simulink model "Brat_Robotic"  (R2022b)
settings: Solver=VariableStepAuto  StartTime=0.0  StopTime=timp  MaxStep=0.01  RelTol=1e-3
InitFcn:
  | %Elements lengths cm
  |     l1 = 24;
  |     l2 = 24;
  |     l3 = 20;
  |     l4 = 24;
  |     l5 = 10;
  |     l6 = 8;
  |     l7= 7;
  | 
  |     %sim time
  |     %timp=10;
  | 
  |     D1 = input_cupla_1/100;
  |     D2 = input_cupla_2*pi/180;
  |     D3 = input_cupla_3*pi/180;
  |     D4 = input_cupla_4/100;
  |     D5 = input_cupla_5*pi/180;
  |     D6 = input_cupla_6/100;
  |     D7 = input_cupla_7/100;
  | 
  |     %{
  |     D1 = 0.04;
  |     D2 = pi/3;
  |     D3 = -pi/5;
  |     D4 = 0.06;
  |     D5 = pi/8;
  |     D6 = 0.02;
  |     D7 = 0.02;
  | 
  |     prompt="Folositi comenzile default: ";
  |     default = input(prompt);
  | 
  |     if (default == 0)
  | 
  | 
  |     prompt="Cupla 1 (translatie):";
  |     D1 = input(prompt);
  |     prompt="Cupla 2 (rotatie):";
  |     D2 = input(prompt);
  |     prompt="Cupla 3 (rotatie):";
  |     D3 = input(prompt);
  |     prompt="Cupla 4 (translatie):";
  |     D4 = input(prompt);
  |     prompt="Cupla 5 (rotatie):";
  |     D5 = input(prompt);
  |     prompt="Cupla 6 (translatie):";
  |     D6 = input(prompt);
  |     prompt="Cupla 7 (translatie):";
  |     D7 = input(prompt);
  | 
  |     end
  |     %}
  | 
  |     t=0:0.01:timp;
  |     n=length(t);
  | 
  |     %generam vectori linie egali distribuiti cu n elemente
  |     D1_v=linspace(0,D1,n);
  |     D2_v=linspace(0,D2,n);
  |     D3_v=linspace(0,D3,n);
  | ... (+14 lines)
StopFcn:
  | %close all;
  | 
  | %t=0:0.01:timp;
  | 
  | %forte totale in fiecare cupla pe cele 3 axe in fiecare moment de timp
  | %{
  | forta_cupla_1=squeeze(out.forta_tot_cupla1);
  | forta_cupla_2=squeeze(forta_tot_cupla2);
  | forta_cupla_3=squeeze(forta_tot_cupla3);
  | forta_cupla_4=squeeze(forta_tot_cupla4);
  | forta_cupla_5=squeeze(forta_tot_cupla5);
  | forta_cupla_6=squeeze(forta_tot_cupla6);
  | forta_cupla_7=squeeze(forta_tot_cupla7);
  | 
  | momt_cupla1=squeeze(moment_tot_cupla1);
  | momt_cupla2=squeeze(moment_tot_cupla2);
  | momt_cupla3=squeeze(moment_tot_cupla3);
  | momt_cupla4=squeeze(moment_tot_cupla4);
  | momt_cupla5=squeeze(moment_tot_cupla5);
  | momt_cupla6=squeeze(moment_tot_cupla6);
  | momt_cupla7=squeeze(moment_tot_cupla7);
  | 
  | x_traiectorie=squeeze(x_cupla5(1,1,:));
  | y_traiectorie=squeeze(y_cupla5(1,1,:));
  | z_traiectorie=squeeze(z_cupla5(1,1,:));
  | 
  | 
  | figure
  | plot3(x_traiectorie(:,1),y_traiectorie(:,1),-z_traiectorie(:,1),'*k');
  | xlabel('x')
  | ylabel('y')
  | zlabel('z')
  | title("Traiectoria efectorului final")
  | grid on
  | 
  | nr_cupla = -1;
  | 
  | while nr_cupla ~= 0
  | 
  | prompt="Introduceti numarul cuplei despre care vreti sa aflati torsorul: ";
  | nr_cupla = input(prompt);
  | 
  | switch nr_cupla
  | 
  |     case 0
  |         disp('Exited')
  |     case 1
  |         plot_informatii_cupla(forta_cupla_1, momt_cupla1, t);
  |     case 2
  |         plot_informatii_cupla(forta_cupla_2, momt_cupla2, t);
  |     case 3
  |         plot_informatii_cupla(forta_cupla_3, momt_cupla3, t);
  |     case 4
  |         plot_informatii_cupla(forta_cupla_4, momt_cupla4, t);
  |     case 5
  |         plot_informatii_cupla(forta_cupla_5, momt_cupla5, t);
  |     case 6
  |         plot_informatii_cupla(forta_cupla_6, momt_cupla6, t);
  |     case 7
  |         plot_informatii_cupla(forta_cupla_7, momt_cupla7, t);
  | ... (+6 lines)
undefined symbols (not defined in the file or in its folder): X, Y, Z
libraries: sm_lib x35, nesl_utility x25, simulink x14
(part 2 of 2)

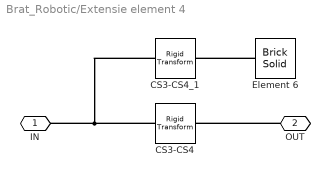
== system Brat_Robotic/Extensie element 4 ==
  CS3-CS4 : sm_lib/Frames and Transforms/Rigid Transform  TranslationMethod=StandardAxis  TranslationStandardOffset=l3  TranslationLengthUnit=cm  TranslationStandardAxis=+X  TranslationCartesianOffset=[0 0 0]  TranslationROffset=0  TranslationROffsetUnits=m  TranslationZOffset=0  TranslationZOffsetUnits=m  TranslationThetaOffset=0  TranslationThetaOffsetUnits=deg  RotationMethod=StandardAxis  RotationAngleUnits=deg  RotationStandardAxis=+Y  RotationAngle=90  RotationArbitraryAxis=[0 0 1]  FollAlignAxisA=+X  BaseAlignAxisA=+Y  FollAlignAxisB=+Y  BaseAlignAxisB=+Z  RotationSequenceAxes=FollowerAxes  RotationSequence=XYX  RotationSequenceAngles=[0 0 0]  RotationSequenceAnglesUnits=deg  RotationMatrix=[1 0 0; 0 1 0; 0 0 1]  Quaternion=[1 0 0 0]
  CS3-CS4_1 : sm_lib/Frames and Transforms/Rigid Transform  TranslationMethod=StandardAxis  TranslationStandardOffset=l3  TranslationLengthUnit=cm  TranslationStandardAxis=+X  TranslationCartesianOffset=[0 0 0]  TranslationROffset=0  TranslationROffsetUnits=m  TranslationZOffset=0  TranslationZOffsetUnits=m  TranslationThetaOffset=0  TranslationThetaOffsetUnits=deg  RotationMethod=StandardAxis  RotationAngleUnits=deg  RotationStandardAxis=+Y  RotationAngle=90  RotationArbitraryAxis=[0 0 1]  FollAlignAxisA=+X  BaseAlignAxisA=+Y  FollAlignAxisB=+Y  BaseAlignAxisB=+Z  RotationSequenceAxes=FollowerAxes  RotationSequence=XYX  RotationSequenceAngles=[0 0 0]  RotationSequenceAnglesUnits=deg  RotationMatrix=[1 0 0; 0 1 0; 0 0 1]  Quaternion=[1 0 0 0]
  Element 6 : sm_lib/Body Elements/Brick Solid  GraphicAmbientColor=[0.15 0.15 0.15 1.0]  BasedOnType=Density  BrickDimensions=[8 8 D4*100+0.01]  BrickDimensionUnits=cm  CenterOfMass=[0 0 0]  CenterOfMassUnits=m  GraphicDiffuseColor=[1.0 0.0 0.2]  Density=1000  DensityUnits=kg/m^3  DoExposeReferenceFrame=off  GraphicEmissiveColor=[0.0 0.0 0.0 1.0]  ExportEntireGeometry=off  SerializedFrames=<Frames><Frame><Id>Frame1</Id><Value><Name>F1</Name><Origin><Source>GeometricFeature</Source><FeatureName>-z surface</FeatureName></Origin><PrimaryAxis><DefinedDirection>+Z</DefinedDirection><Source>ReferenceFrame</Source><SourceDirection>+Z</SourceDirection><FeatureName></FeatureName></PrimaryAxis><SecondaryAxis><DefinedDirection>+X</DefinedDirection><Source>ReferenceFrame</Source><SourceDirection>+X</SourceDirection><FeatureName></FeatureName></SecondaryAxis></Value></Frame></Frames>  MarkerShape=Sphere  MarkerSize=10  GraphicType=FromGeometry  InertiaType=CalculateFromGeometry  Mass=1  MassUnits=kg  MomentsOfInertia=[1 1 1]  MomentsOfInertiaUnits=kg*m^2  GraphicOpacity=1.0  ProductsOfInertia=[0 0 0]  ProductsOfInertiaUnits=kg*m^2  GraphicShininess=75  GraphicSpecularColor=[0.5 0.5 0.5 1.0]  GraphicVisPropType=SimpleVisualProperties
  IN : PMIOPort  Side=Left
  OUT : PMIOPort  Port=2  Side=Right
  connections:
  CS3-CS4/LConn1 -- CS3-CS4_1/LConn1 -- IN/RConn1
  Element 6/LConn1 -- CS3-CS4_1/RConn1
  OUT/RConn1 -- CS3-CS4/RConn1

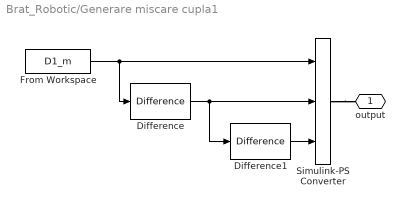
== system Brat_Robotic/Generare miscare cupla1 ==
  Difference : simulink/Discrete/Difference  ICPrevInput=0.0  OutMin=[]  OutMax=[]  OutDataType=fixdt(1, 16)  OutScaling=2^-10  DoSatur=off
  Difference1 : simulink/Discrete/Difference  ICPrevInput=0.0  OutMin=[]  OutMax=[]  OutDataType=fixdt(1, 16)  OutScaling=2^-10  DoSatur=off
  From Workspace : FromWorkspace  VariableName=D1_m
  Simulink-PS Converter : nesl_utility/Simulink-PS Converter  PhysicalDomain=network_engine_domain  SubClassName=ps_input  LeftPortType=input  RightPortType=output  PseudoPeriodic=off  Frequencies=[]  NoiseDistribution=none  NoiseParameters=[]  Unit=1  AffineConversion=off  FilteringAndDerivatives=provide  SimscapeFilterOrder=1  InputFilterTimeConstant=0.001  UdotUserProvided=2
  output : PMIOPort  Side=Right
  wires:
  From Workspace/1 -> Difference/1, Simulink-PS Converter/1
  Difference1/1 -> Simulink-PS Converter/3
  Difference/1 -> Difference1/1, Simulink-PS Converter/2
  connections:
  Simulink-PS Converter/RConn1 -- output/RConn1

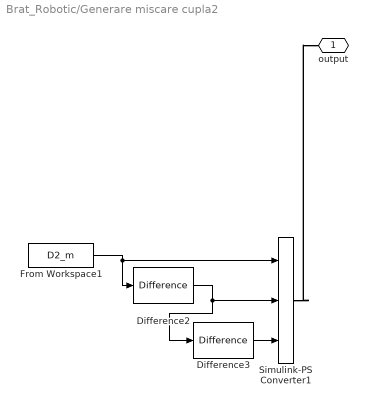
== system Brat_Robotic/Generare miscare cupla2 ==
  Difference2 : simulink/Discrete/Difference  ICPrevInput=0.0  OutMin=[]  OutMax=[]  OutDataType=fixdt(1, 16)  OutScaling=2^-10  DoSatur=off
  Difference3 : simulink/Discrete/Difference  ICPrevInput=0.0  OutMin=[]  OutMax=[]  OutDataType=fixdt(1, 16)  OutScaling=2^-10  DoSatur=off
  From Workspace1 : FromWorkspace  VariableName=D2_m
  Simulink-PS Converter1 : nesl_utility/Simulink-PS Converter  PhysicalDomain=network_engine_domain  SubClassName=ps_input  LeftPortType=input  RightPortType=output  PseudoPeriodic=off  Frequencies=[]  NoiseDistribution=none  NoiseParameters=[]  Unit=1  AffineConversion=off  FilteringAndDerivatives=provide  SimscapeFilterOrder=1  InputFilterTimeConstant=0.001  UdotUserProvided=2
  output : PMIOPort  Side=Right
  wires:
  Difference2/1 -> Difference3/1, Simulink-PS Converter1/2
  From Workspace1/1 -> Difference2/1, Simulink-PS Converter1/1
  Difference3/1 -> Simulink-PS Converter1/3
  connections:
  Simulink-PS Converter1/RConn1 -- output/RConn1

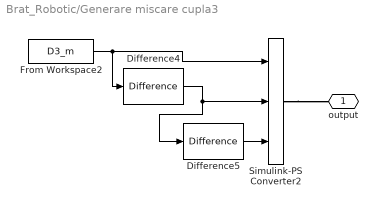
== system Brat_Robotic/Generare miscare cupla3 ==
  Difference4 : simulink/Discrete/Difference  ICPrevInput=0.0  OutMin=[]  OutMax=[]  OutDataType=fixdt(1, 16)  OutScaling=2^-10  DoSatur=off
  Difference5 : simulink/Discrete/Difference  ICPrevInput=0.0  OutMin=[]  OutMax=[]  OutDataType=fixdt(1, 16)  OutScaling=2^-10  DoSatur=off
  From Workspace2 : FromWorkspace  VariableName=D3_m
  Simulink-PS Converter2 : nesl_utility/Simulink-PS Converter  PhysicalDomain=network_engine_domain  SubClassName=ps_input  LeftPortType=input  RightPortType=output  PseudoPeriodic=off  Frequencies=[]  NoiseDistribution=none  NoiseParameters=[]  Unit=1  AffineConversion=off  FilteringAndDerivatives=provide  SimscapeFilterOrder=1  InputFilterTimeConstant=0.001  UdotUserProvided=2
  output : PMIOPort  Side=Right
  wires:
  Difference4/1 -> Difference5/1, Simulink-PS Converter2/2
  From Workspace2/1 -> Simulink-PS Converter2/1, Difference4/1
  Difference5/1 -> Simulink-PS Converter2/3
  connections:
  Simulink-PS Converter2/RConn1 -- output/RConn1

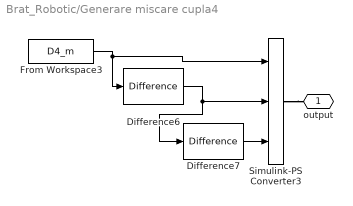
== system Brat_Robotic/Generare miscare cupla4 ==
  Difference6 : simulink/Discrete/Difference  ICPrevInput=0.0  OutMin=[]  OutMax=[]  OutDataType=fixdt(1, 16)  OutScaling=2^-10  DoSatur=off
  Difference7 : simulink/Discrete/Difference  ICPrevInput=0.0  OutMin=[]  OutMax=[]  OutDataType=fixdt(1, 16)  OutScaling=2^-10  DoSatur=off
  From Workspace3 : FromWorkspace  VariableName=D4_m
  Simulink-PS Converter3 : nesl_utility/Simulink-PS Converter  PhysicalDomain=network_engine_domain  SubClassName=ps_input  LeftPortType=input  RightPortType=output  PseudoPeriodic=off  Frequencies=[]  NoiseDistribution=none  NoiseParameters=[]  Unit=1  AffineConversion=off  FilteringAndDerivatives=provide  SimscapeFilterOrder=1  InputFilterTimeConstant=0.001  UdotUserProvided=2
  output : PMIOPort  Side=Right
  wires:
  Difference6/1 -> Difference7/1, Simulink-PS Converter3/2
  From Workspace3/1 -> Difference6/1, Simulink-PS Converter3/1
  Difference7/1 -> Simulink-PS Converter3/3
  connections:
  Simulink-PS Converter3/RConn1 -- output/RConn1

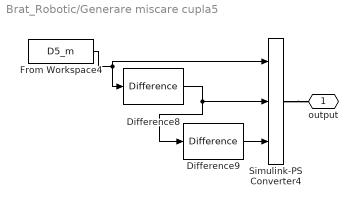
== system Brat_Robotic/Generare miscare cupla5 ==
  Difference8 : simulink/Discrete/Difference  ICPrevInput=0.0  OutMin=[]  OutMax=[]  OutDataType=fixdt(1, 16)  OutScaling=2^-10  DoSatur=off
  Difference9 : simulink/Discrete/Difference  ICPrevInput=0.0  OutMin=[]  OutMax=[]  OutDataType=fixdt(1, 16)  OutScaling=2^-10  DoSatur=off
  From Workspace4 : FromWorkspace  VariableName=D5_m
  Simulink-PS Converter4 : nesl_utility/Simulink-PS Converter  PhysicalDomain=network_engine_domain  SubClassName=ps_input  LeftPortType=input  RightPortType=output  PseudoPeriodic=off  Frequencies=[]  NoiseDistribution=none  NoiseParameters=[]  Unit=1  AffineConversion=off  FilteringAndDerivatives=provide  SimscapeFilterOrder=1  InputFilterTimeConstant=0.001  UdotUserProvided=2
  output : PMIOPort  Side=Right
  wires:
  From Workspace4/1 -> Simulink-PS Converter4/1, Difference8/1
  Difference9/1 -> Simulink-PS Converter4/3
  Difference8/1 -> Difference9/1, Simulink-PS Converter4/2
  connections:
  Simulink-PS Converter4/RConn1 -- output/RConn1

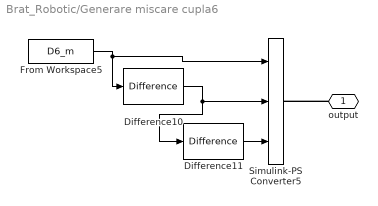
== system Brat_Robotic/Generare miscare cupla6 ==
  Difference10 : simulink/Discrete/Difference  ICPrevInput=0.0  OutMin=[]  OutMax=[]  OutDataType=fixdt(1, 16)  OutScaling=2^-10  DoSatur=off
  Difference11 : simulink/Discrete/Difference  ICPrevInput=0.0  OutMin=[]  OutMax=[]  OutDataType=fixdt(1, 16)  OutScaling=2^-10  DoSatur=off
  From Workspace5 : FromWorkspace  VariableName=D6_m
  Simulink-PS Converter5 : nesl_utility/Simulink-PS Converter  PhysicalDomain=network_engine_domain  SubClassName=ps_input  LeftPortType=input  RightPortType=output  PseudoPeriodic=off  Frequencies=[]  NoiseDistribution=none  NoiseParameters=[]  Unit=1  AffineConversion=off  FilteringAndDerivatives=provide  SimscapeFilterOrder=1  InputFilterTimeConstant=0.001  UdotUserProvided=2
  output : PMIOPort  Side=Right
  wires:
  Difference10/1 -> Difference11/1, Simulink-PS Converter5/2
  From Workspace5/1 -> Difference10/1, Simulink-PS Converter5/1
  Difference11/1 -> Simulink-PS Converter5/3
  connections:
  output/RConn1 -- Simulink-PS Converter5/RConn1

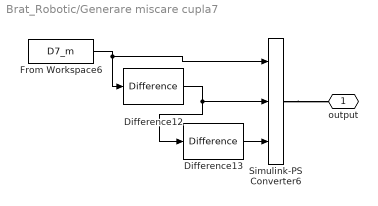
== system Brat_Robotic/Generare miscare cupla7 ==
  Difference12 : simulink/Discrete/Difference  ICPrevInput=0.0  OutMin=[]  OutMax=[]  OutDataType=fixdt(1, 16)  OutScaling=2^-10  DoSatur=off
  Difference13 : simulink/Discrete/Difference  ICPrevInput=0.0  OutMin=[]  OutMax=[]  OutDataType=fixdt(1, 16)  OutScaling=2^-10  DoSatur=off
  From Workspace6 : FromWorkspace  VariableName=D7_m
  Simulink-PS Converter6 : nesl_utility/Simulink-PS Converter  PhysicalDomain=network_engine_domain  SubClassName=ps_input  LeftPortType=input  RightPortType=output  PseudoPeriodic=off  Frequencies=[]  NoiseDistribution=none  NoiseParameters=[]  Unit=1  AffineConversion=off  FilteringAndDerivatives=provide  SimscapeFilterOrder=1  InputFilterTimeConstant=0.001  UdotUserProvided=2
  output : PMIOPort  Side=Right
  wires:
  Difference13/1 -> Simulink-PS Converter6/3
  From Workspace6/1 -> Difference12/1, Simulink-PS Converter6/1
  Difference12/1 -> Difference13/1, Simulink-PS Converter6/2
  connections:
  Simulink-PS Converter6/RConn1 -- output/RConn1

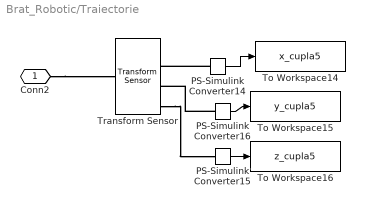
== system Brat_Robotic/Traiectorie ==
  PS-Simulink Converter14 : nesl_utility/PS-Simulink Converter  PhysicalDomain=network_engine_domain  SubClassName=ps_output  LeftPortType=input  RightPortType=output  PseudoPeriodic=off  Frequencies=[]  VectorFormat=inherit  Unit=inherit  AffineConversion=off
  PS-Simulink Converter15 : nesl_utility/PS-Simulink Converter  PhysicalDomain=network_engine_domain  SubClassName=ps_output  LeftPortType=input  RightPortType=output  PseudoPeriodic=off  Frequencies=[]  VectorFormat=inherit  Unit=inherit  AffineConversion=off
  PS-Simulink Converter16 : nesl_utility/PS-Simulink Converter  PhysicalDomain=network_engine_domain  SubClassName=ps_output  LeftPortType=input  RightPortType=output  PseudoPeriodic=off  Frequencies=[]  VectorFormat=inherit  Unit=inherit  AffineConversion=off
  To Workspace14 : ToWorkspace  VariableName=x_cupla5  SampleTime=-1
  To Workspace15 : ToWorkspace  VariableName=y_cupla5  SampleTime=-1
  To Workspace16 : ToWorkspace  VariableName=z_cupla5  SampleTime=-1
  Transform Sensor : sm_lib/Frames and Transforms/Transform Sensor  MeasurementFrame=World  SenseAngle=off  SenseAxis=off  SenseQ=off  SenseR=off  SenseRotationSequence=off  RotationSequence=XYX  SenseOmegaX=off  SenseOmegaY=off  SenseOmegaZ=off  SenseQDot=off  SenseRDot=off  SenseAlphaX=off  SenseAlphaY=off  SenseAlphaZ=off  SenseQDDot=off  SenseRDDot=off  SenseX=on  SenseY=on  SenseZ=on  SenseRad=off  SenseAzim=off  SenseDist=off  SenseInc=off  SenseXDot=off  SenseYDot=off  SenseZDot=off  SenseRadDot=off  SenseAzimDot=off  SenseDistDot=off  SenseIncDot=off  SenseXDDot=off  SenseYDDot=off  SenseZDDot=off  SenseRadDDot=off  SenseAzimDDot=off  SenseDistDDot=off  SenseIncDDot=off
  Conn2 : PMIOPort  Side=Left
  wires:
  PS-Simulink Converter16/1 -> To Workspace15/1
  PS-Simulink Converter14/1 -> To Workspace14/1
  PS-Simulink Converter15/1 -> To Workspace16/1
  connections:
  PS-Simulink Converter16/LConn1 -- Transform Sensor/RConn3
  PS-Simulink Converter14/LConn1 -- Transform Sensor/RConn2
  Transform Sensor/RConn4 -- PS-Simulink Converter15/LConn1
  Conn2/RConn1 -- Transform Sensor/LConn1
